simulink subsystem "IKS02A1_Error_Detected"  (R2024b)
settings: Solver=VariableStepAuto  StartTime=0.0  StopTime=10.0  RelTol=1e-3
settings Model: Creator=JesseJabezArendse  LastModifiedBy=JesseJabezArendse

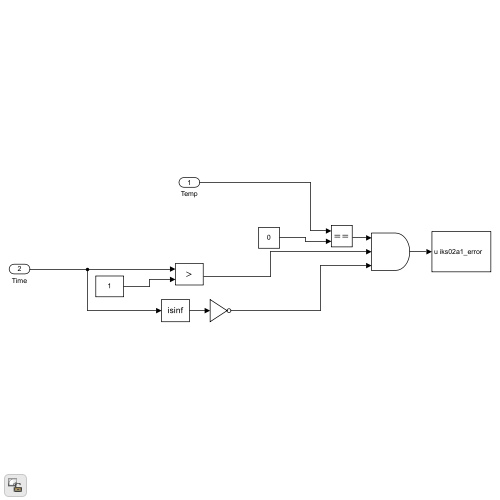
[thumbnail: Simulink's stored preview of the top-level diagram]
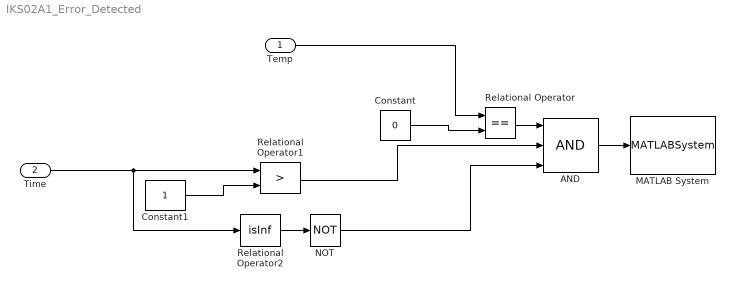
== system IKS02A1_Error_Detected ==
  Temp : Inport
  Time : Inport  Port=2
  AND : Logic  Inputs=3  IconShape=distinctive  AllPortsSameDT=off  OutDataTypeStr=boolean
  Constant : Constant  Value=0
  Constant1 : Constant
  MATLAB System : MATLABSystem  System=iks02a1_error  SimulateUsing=Code generation
      mask Type: iks02a1_error
      mask Display:
      | disp('iks02a1_error');
      | port_label('input',1,'u');
  NOT : Logic  Operator=NOT  IconShape=distinctive  AllPortsSameDT=off  OutDataTypeStr=boolean
  Relational Operator : RelationalOperator  Operator===  OutDataTypeStr=boolean  RndMeth=Simplest  InputSameDT=off
  Relational Operator1 : RelationalOperator  Operator=>  OutDataTypeStr=boolean  RndMeth=Simplest  InputSameDT=off
  Relational Operator2 : RelationalOperator  Operator=isInf  OutDataTypeStr=boolean  RndMeth=Simplest  InputSameDT=off
  wires:
  Temp/1 -> Relational Operator/1
  AND/1 -> MATLAB System/1
  Constant/1 -> Relational Operator/2
  Relational Operator/1 -> AND/1
  Constant1/1 -> Relational Operator1/2
  Time/1 -> Relational Operator1/1, Relational Operator2/1
  Relational Operator1/1 -> AND/2
  Relational Operator2/1 -> NOT/1
  NOT/1 -> AND/3
